simulink model "DynamicModel_DiferentialDrive"  (R2018a)
settings: Solver=ode4  StartTime=0.0  StopTime=100  FixedStep=0.01  RelTol=1e-3
libraries: simulink x1
settings Model: Creator=Yuri  LastModifiedBy=Yuri
settings SolverCC: AlgebraicLoopSolver=LineSearch

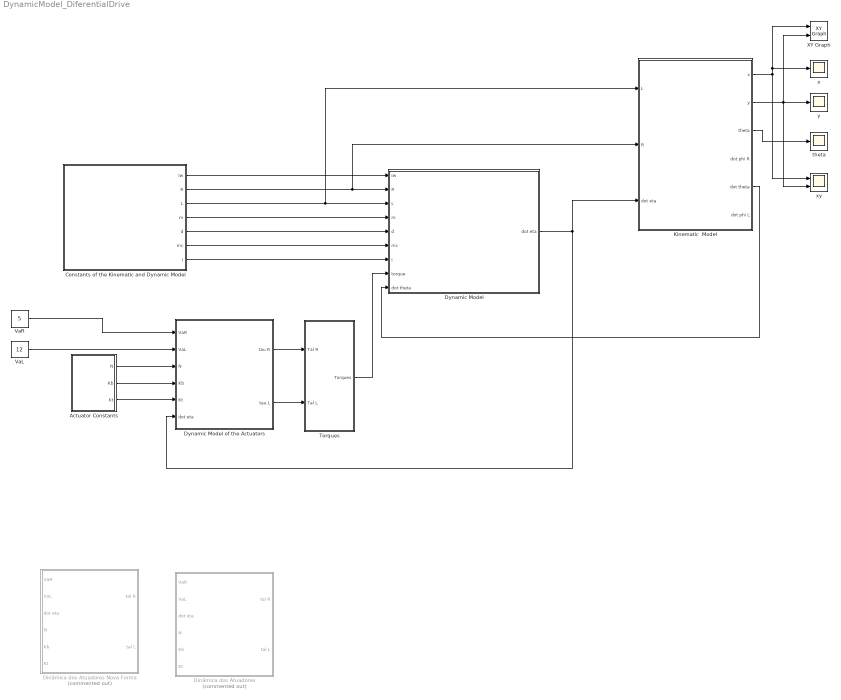
== system DynamicModel_DiferentialDrive ==
  Actuator Constants : Subsystem
  Constants of the Kinematic and Dynamic Model : Subsystem
  "Dinâmica dos Atuadores " : Subsystem  Commented=on
  Dinâmica dos Atuadores Nova Forma : Subsystem  Commented=on
  Dynamic Model : Subsystem
  Dynamic Model of the Actuators : Subsystem
  Kinematic  Model : Subsystem
  Torques : Subsystem
  VaL : Constant  Value=12
  VaR : Constant  Value=5
  XY Graph : simulink/Sinks/XY Graph  xmin=-25  xmax=25  ymin=-25  ymax=25  st=-1
  "theta " : Scope
  x : Scope
  xy : Scope  NumInputPorts=2
  y : Scope
  wires:
  Torques/1("Torques ") -> Dynamic Model/8(torque)
  Kinematic  Model/3(theta) -> "theta "/1
  Kinematic  Model/1(x) -> xy/1, XY Graph/1, x/1
  Kinematic  Model/2(y) -> xy/2, XY Graph/2, y/1
  Kinematic  Model/5(dot theta) -> Dynamic Model/9(dot theta)
  Dynamic Model/1(dot eta) -> Dynamic Model of the Actuators/6(dot eta), Kinematic  Model/3(dot eta)
  VaR/1 -> Dynamic Model of the Actuators/1(VaR)
  VaL/1 -> Dynamic Model of the Actuators/2(VaL)
  Dynamic Model of the Actuators/1(tau R) -> Torques/1(Tal R)
  Dynamic Model of the Actuators/2(tau L) -> Torques/2(Tal L)
  Constants of the Kinematic and Dynamic Model/5("d ") -> Dynamic Model/5(d)
  Constants of the Kinematic and Dynamic Model/3("L ") -> Kinematic  Model/1(L), Dynamic Model/3(L)
  Constants of the Kinematic and Dynamic Model/2("R ") -> Kinematic  Model/2(R), Dynamic Model/2(R)
  Constants of the Kinematic and Dynamic Model/6("mc ") -> Dynamic Model/6(mc)
  Constants of the Kinematic and Dynamic Model/1("Iw ") -> Dynamic Model/1(Iw)
  Constants of the Kinematic and Dynamic Model/4("m ") -> Dynamic Model/4(m)
  Actuator Constants/1(N) -> Dynamic Model of the Actuators/3("N ")
  Actuator Constants/3("Kt ") -> Dynamic Model of the Actuators/5("Kt ")
  Actuator Constants/2("Kb ") -> Dynamic Model of the Actuators/4("Kb ")
  Constants of the Kinematic and Dynamic Model/7("I ") -> Dynamic Model/7(I)

== system DynamicModel_DiferentialDrive/Actuator Constants ==
  Kb : Constant  Value=0.029
  Kt : Constant  Value=0.023
  "N  " : Constant  Value=38.3
  N : Outport
  "Kb " : Outport  Port=2
  "Kt " : Outport  Port=3
  wires:
  Kb/1 -> "Kb "/1
  Kt/1 -> "Kt "/1
  "N  "/1 -> N/1

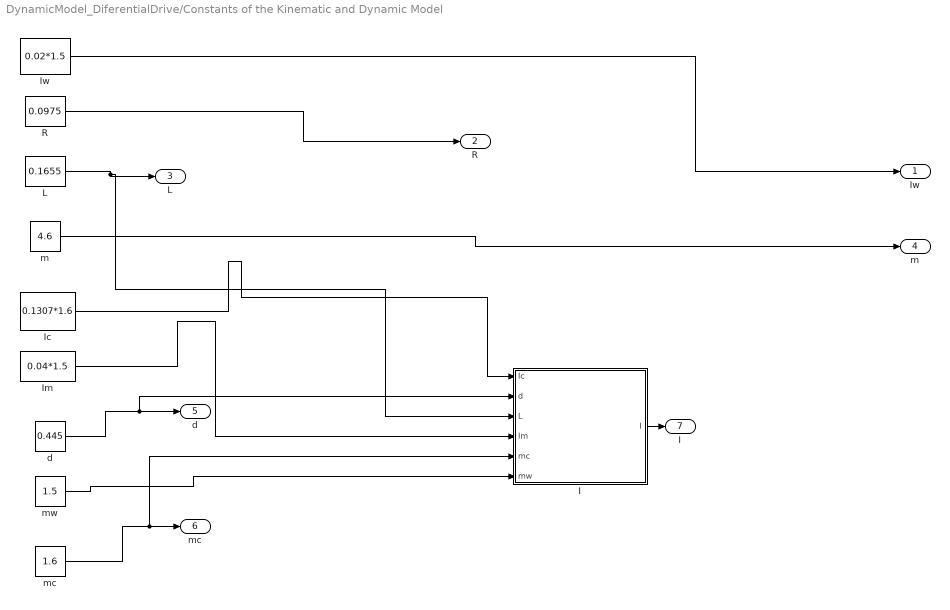
== system DynamicModel_DiferentialDrive/Constants of the Kinematic and Dynamic Model ==
  I : Subsystem
  Ic : Constant  Value=0.1307*1.6
  Im : Constant  Value=0.04*1.5
  Iw : Constant  Value=0.02*1.5
  L : Constant  Value=0.1655  VectorParams1D=off
  R : Constant  Value=0.0975
  d : Constant  Value=0.445
  m : Constant  Value=4.6
  mc : Constant  Value=1.6
  mw : Constant  Value=1.5
  "Iw " : Outport
  "R " : Outport  Port=2
  "L " : Outport  Port=3
  "m " : Outport  Port=4
  "d " : Outport  Port=5
  "mc " : Outport  Port=6
  "I " : Outport  Port=7
  wires:
  Im/1 -> I/4(Im)
  Ic/1 -> I/1(Ic)
  d/1 -> I/2(d), "d "/1
  R/1 -> "R "/1
  Iw/1 -> "Iw "/1
  mw/1 -> I/6(mw)
  m/1 -> "m "/1
  mc/1 -> I/5(mc), "mc "/1
  L/1 -> I/3(L), "L "/1
  I/1(I) -> "I "/1

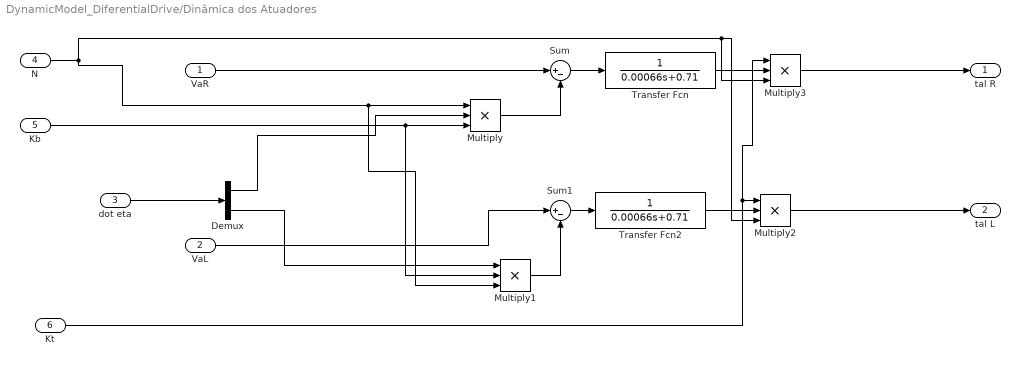
== system DynamicModel_DiferentialDrive/Dinâmica dos Atuadores  ==
  VaR : Inport
  VaL : Inport  Port=2
  dot eta : Inport  Port=3
  "N " : Inport  Port=4
  "Kb " : Inport  Port=5
  "Kt " : Inport  Port=6
  Demux : Demux  Outputs=2
  Multiply{,1..3} (4 alike) : Product  Inputs=3
  Sum : Sum  Inputs=|+-
  Sum1 : Sum  Inputs=|+-
  Transfer Fcn : TransferFcn  Denominator=[0.00066 0.71]
  Transfer Fcn2 : TransferFcn  Denominator=[0.00066 0.71]
  tal R : Outport
  tal L : Outport  Port=2
  wires:
  VaR/1 -> Sum/1
  Sum/1 -> Transfer Fcn/1
  Demux/1 -> Multiply/2
  VaL/1 -> Sum1/1
  Sum1/1 -> Transfer Fcn2/1
  Multiply1/1 -> Sum1/2
  dot eta/1 -> Demux/1
  "N "/1 -> Multiply1/3, Multiply/1, Multiply2/3, Multiply3/3
  "Kb "/1 -> Multiply1/2, Multiply/3
  Demux/2 -> Multiply1/1
  Multiply/1 -> Sum/2
  Transfer Fcn2/1 -> Multiply2/2
  Transfer Fcn/1 -> Multiply3/2
  "Kt "/1 -> Multiply3/1, Multiply2/1
  Multiply3/1 -> tal R/1
  Multiply2/1 -> tal L/1

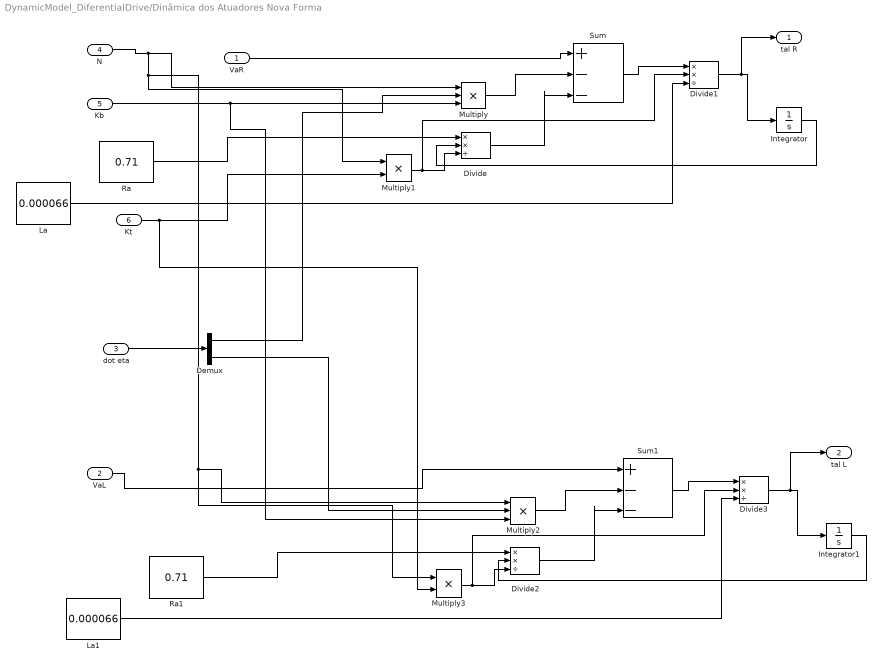
== system DynamicModel_DiferentialDrive/Dinâmica dos Atuadores Nova Forma ==
  VaR : Inport
  VaL : Inport  Port=2
  dot eta : Inport  Port=3
  "N " : Inport  Port=4
  "Kb " : Inport  Port=5
  "Kt " : Inport  Port=6
  Demux : Demux  Outputs=2
  Divide{,1..3} (4 alike) : Product  Inputs=**/
  Integrator : Integrator
  Integrator1 : Integrator
  La : Constant  Value=0.000066
  La1 : Constant  Value=0.000066
  Multiply : Product  Inputs=3
  Multiply1 : Product
  Multiply2 : Product  Inputs=3
  Multiply3 : Product
  Ra : Constant  Value=0.71
  Ra1 : Constant  Value=0.71
  Sum : Sum  Inputs=|+--
  Sum1 : Sum  Inputs=|+--
  tal R : Outport
  tal L : Outport  Port=2
  wires:
  VaR/1 -> Sum/1
  Demux/1 -> Multiply/2
  dot eta/1 -> Demux/1
  Multiply/1 -> Sum/2
  "Kt "/1 -> Multiply3/2, Multiply1/2
  Ra/1 -> Divide/1
  Multiply1/1 -> Divide1/2, Divide/3
  Integrator/1 -> Divide/2
  Divide/1 -> Sum/3
  Divide1/1 -> tal R/1, Integrator/1
  Sum/1 -> Divide1/1
  La/1 -> Divide1/3
  Divide3/1 -> tal L/1, Integrator1/1
  VaL/1 -> Sum1/1
  Demux/2 -> Multiply2/2
  Sum1/1 -> Divide3/1
  Multiply2/1 -> Sum1/2
  Divide2/1 -> Sum1/3
  "Kb "/1 -> Multiply2/3, Multiply/3
  Ra1/1 -> Divide2/1
  Integrator1/1 -> Divide2/2
  "N "/1 -> Multiply3/1, Multiply2/1, Multiply1/1, Multiply/1
  La1/1 -> Divide3/3
  Multiply3/1 -> Divide3/2, Divide2/3

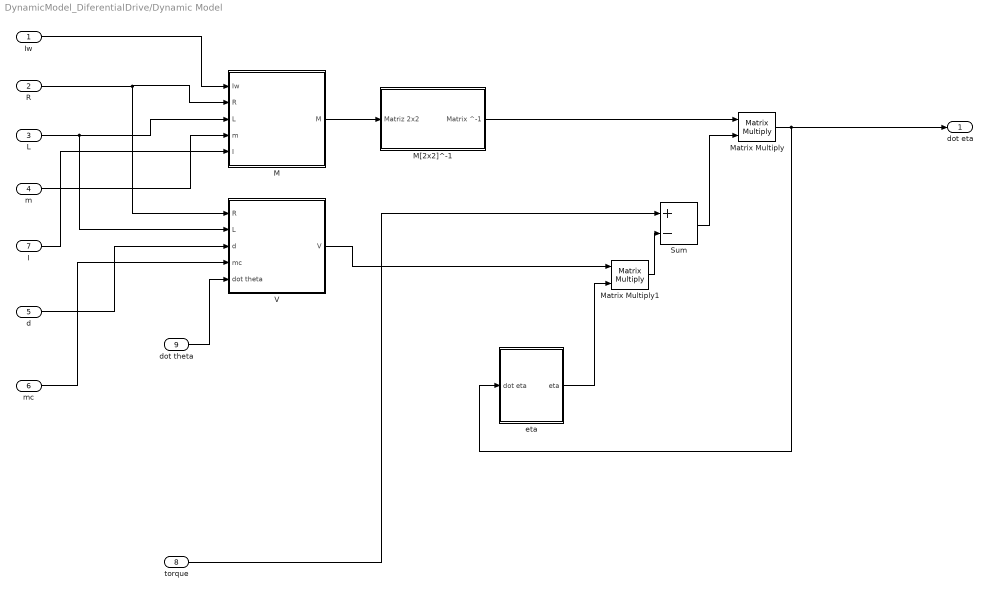
== system DynamicModel_DiferentialDrive/Dynamic Model ==
  Iw : Inport
  R : Inport  Port=2
  L : Inport  Port=3
  m : Inport  Port=4
  d : Inport  Port=5
  mc : Inport  Port=6
  I : Inport  Port=7
  torque : Inport  Port=8
  dot theta : Inport  Port=9
  " eta" : Subsystem
  M : Subsystem
  M[2x2]^-1 : Subsystem
  Matrix Multiply : Product  Multiplication=Matrix(*)
  Matrix Multiply1 : Product  Multiplication=Matrix(*)
  Sum : Sum  Inputs=+-
  V : Subsystem
  dot eta : Outport
  wires:
  Matrix Multiply1/1 -> Sum/2
  Sum/1 -> Matrix Multiply/2
  " eta"/1("eta ") -> Matrix Multiply1/2
  M[2x2]^-1/1(Matrix ^-1) -> Matrix Multiply/1
  Matrix Multiply/1 -> " eta"/1(dot eta), dot eta/1
  torque/1 -> Sum/1
  L/1 -> V/2(L), M/3(L)
  mc/1 -> V/4(mc)
  R/1 -> M/2(R), V/1(R)
  dot theta/1 -> V/5(dot theta)
  Iw/1 -> M/1(Iw)
  I/1 -> M/5(I)
  m/1 -> M/4(m)
  d/1 -> V/3(d)
  M/1(M) -> M[2x2]^-1/1("Matriz 2x2 ")
  V/1(V) -> Matrix Multiply1/1

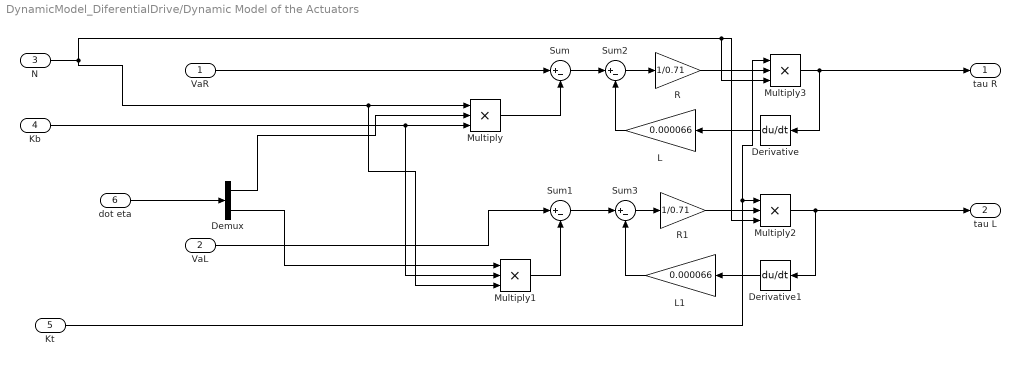
== system DynamicModel_DiferentialDrive/Dynamic Model of the Actuators ==
  VaR : Inport
  VaL : Inport  Port=2
  "N " : Inport  Port=3
  "Kb " : Inport  Port=4
  "Kt " : Inport  Port=5
  dot eta : Inport  Port=6
  Demux : Demux  Outputs=2
  Derivative : Derivative
  Derivative1 : Derivative
  L : Gain  Gain=0.000066
  L1 : Gain  Gain=0.000066
  Multiply{,1..3} (4 alike) : Product  Inputs=3
  R : Gain  Gain=1/0.71
  R1 : Gain  Gain=1/0.71
  Sum{,1..3} (4 alike) : Sum  Inputs=|+-
  tau R : Outport
  tau L : Outport  Port=2
  wires:
  VaR/1 -> Sum/1
  Sum/1 -> Sum2/1
  Demux/1 -> Multiply/2
  VaL/1 -> Sum1/1
  Multiply1/1 -> Sum1/2
  dot eta/1 -> Demux/1
  "N "/1 -> Multiply1/3, Multiply/1, Multiply2/3, Multiply3/3
  "Kb "/1 -> Multiply1/2, Multiply/3
  Demux/2 -> Multiply1/1
  Multiply/1 -> Sum/2
  R1/1 -> Multiply2/2
  Sum2/1 -> R/1
  "Kt "/1 -> Multiply3/1, Multiply2/1
  Multiply3/1 -> Derivative/1, tau R/1
  Multiply2/1 -> Derivative1/1, tau L/1
  Derivative/1 -> L/1
  L/1 -> Sum2/2
  R/1 -> Multiply3/2
  Sum3/1 -> R1/1
  Sum1/1 -> Sum3/1
  L1/1 -> Sum3/2
  Derivative1/1 -> L1/1

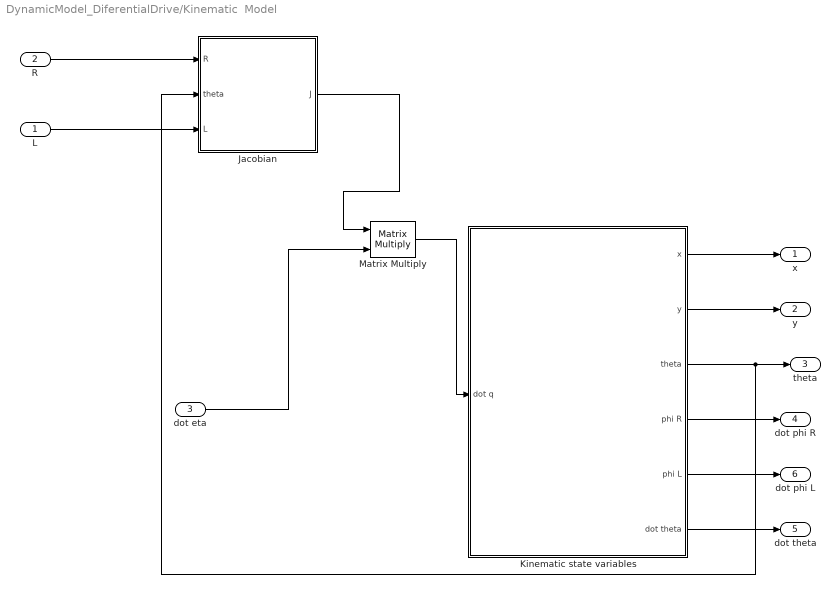
== system DynamicModel_DiferentialDrive/Kinematic  Model ==
  L : Inport
  R : Inport  Port=2
  dot eta : Inport  Port=3
  "Jacobian " : Subsystem
  Kinematic state variables : Subsystem
  Matrix Multiply : Product  Multiplication=Matrix(*)
  x : Outport
  y : Outport  Port=2
  theta : Outport  Port=3
  dot phi R : Outport  Port=4
  dot theta : Outport  Port=5
  dot phi L : Outport  Port=6
  wires:
  Matrix Multiply/1 -> Kinematic state variables/1("dot q ")
  "Jacobian "/1(J) -> Matrix Multiply/1
  Kinematic state variables/5(phi L) -> dot phi L/1
  Kinematic state variables/1(x) -> x/1
  Kinematic state variables/3(theta) -> theta/1, "Jacobian "/2(theta)
  Kinematic state variables/6(dot theta) -> dot theta/1
  R/1 -> "Jacobian "/1(R)
  Kinematic state variables/4(phi R) -> dot phi R/1
  Kinematic state variables/2(y) -> y/1
  L/1 -> "Jacobian "/3(L)
  dot eta/1 -> Matrix Multiply/2

== system DynamicModel_DiferentialDrive/Torques ==
  Tal R : Inport
  Tal L : Inport  Port=2
  Mux : Mux  Inputs=2
  "[2,1]" : Reshape  OutputDimensionality=Customize  OutputDimensions=[2,1]
  "Torques " : Outport
  wires:
  Tal R/1 -> Mux/1
  Tal L/1 -> Mux/2
  Mux/1 -> "[2,1]"/1
  "[2,1]"/1 -> "Torques "/1

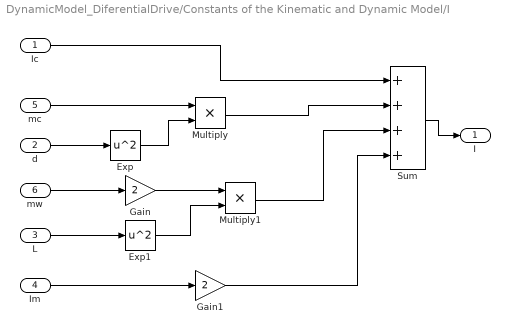
== system DynamicModel_DiferentialDrive/Constants of the Kinematic and Dynamic Model/I ==
  Ic : Inport
  d : Inport  Port=2
  L : Inport  Port=3
  Im : Inport  Port=4
  mc : Inport  Port=5
  mw : Inport  Port=6
  Exp : Math  Operator=square  SaturateOnIntegerOverflow=on
  Exp1 : Math  Operator=square  SaturateOnIntegerOverflow=on
  Gain : Gain  Gain=2
  Gain1 : Gain  Gain=2
  Multiply : Product
  Multiply1 : Product
  Sum : Sum  Inputs=++++
  I : Outport
  wires:
  Ic/1 -> Sum/1
  d/1 -> Exp/1
  Exp/1 -> Multiply/2
  mc/1 -> Multiply/1
  Multiply/1 -> Sum/2
  L/1 -> Exp1/1
  mw/1 -> Gain/1
  Exp1/1 -> Multiply1/2
  Gain/1 -> Multiply1/1
  Multiply1/1 -> Sum/3
  Im/1 -> Gain1/1
  Gain1/1 -> Sum/4
  Sum/1 -> I/1

== system DynamicModel_DiferentialDrive/Dynamic Model/ eta ==
  dot eta : Inport
  Demux : Demux  Outputs=2
  Integrator : Integrator
  Integrator1 : Integrator
  Mux : Mux  Inputs=2
  "[2,1]" : Reshape  OutputDimensionality=Customize  OutputDimensions=[2,1]
  "eta " : Outport
  wires:
  dot eta/1 -> Demux/1
  Demux/1 -> Integrator/1
  Demux/2 -> Integrator1/1
  Integrator1/1 -> Mux/2
  Integrator/1 -> Mux/1
  Mux/1 -> "[2,1]"/1
  "[2,1]"/1 -> "eta "/1

== system DynamicModel_DiferentialDrive/Dynamic Model/M ==
  Iw : Inport
  R : Inport  Port=2
  L : Inport  Port=3
  m : Inport  Port=4
  I : Inport  Port=5
  M11 e M22 : Subsystem
  M12 e M21 : Subsystem
  Mux1 : Mux
  "[1x4] to [2,2]" : Reshape  OutputDimensionality=Customize  OutputDimensions=[2,2]
  M : Outport
  wires:
  Iw/1 -> M11 e M22/1(Iw)
  Mux1/1 -> "[1x4] to [2,2]"/1
  R/1 -> M12 e M21/1(R), M11 e M22/2(R)
  L/1 -> M12 e M21/2(L), M11 e M22/3(L)
  m/1 -> M12 e M21/3("m "), M11 e M22/4("m ")
  I/1 -> M12 e M21/4(I), M11 e M22/5(I)
  M11 e M22/1(M11) -> Mux1/4, Mux1/1
  M12 e M21/1(M12) -> Mux1/3, Mux1/2
  "[1x4] to [2,2]"/1 -> M/1

== system DynamicModel_DiferentialDrive/Dynamic Model/M[2x2]^-1 ==
  "Matriz 2x2 " : Inport
  Demux : Demux
  Gain : Gain  Gain=-1
  Gain1 : Gain  Gain=-1
  Mux : Mux
  Reshape : Reshape  OutputDimensionality=Customize  OutputDimensions=[4,1]
  Reshape1 : Reshape  OutputDimensionality=Customize  OutputDimensions=[2,2]
  Matrix ^-1 : Outport
  wires:
  "Matriz 2x2 "/1 -> Reshape/1
  Demux/1 -> Mux/4
  Demux/4 -> Mux/1
  Demux/2 -> Gain/1
  Gain/1 -> Mux/2
  Demux/3 -> Gain1/1
  Gain1/1 -> Mux/3
  Mux/1 -> Reshape1/1
  Reshape/1 -> Demux/1
  Reshape1/1 -> Matrix ^-1/1

== system DynamicModel_DiferentialDrive/Dynamic Model/V ==
  R : Inport
  L : Inport  Port=2
  d : Inport  Port=3
  mc : Inport  Port=4
  dot theta : Inport  Port=5
  Constant : Constant  Value=0
  Mux1 : Mux
  V12 : Subsystem
  V21 : Subsystem
  "[4x1] to [2,2]" : Reshape  OutputDimensionality=Customize  OutputDimensions=[2,2]
  V : Outport
  wires:
  Constant/1 -> Mux1/4, Mux1/1
  V12/1("V12 ") -> Mux1/2
  V21/1("V21 ") -> Mux1/3
  R/1 -> V21/1(R), V12/1(R)
  L/1 -> V21/2(L), V12/2(L)
  d/1 -> V21/3(d), V12/3(d)
  dot theta/1 -> V21/5(dot theta), V12/5(dot theta)
  mc/1 -> V21/4(mc), V12/4(mc)
  Mux1/1 -> "[4x1] to [2,2]"/1
  "[4x1] to [2,2]"/1 -> V/1

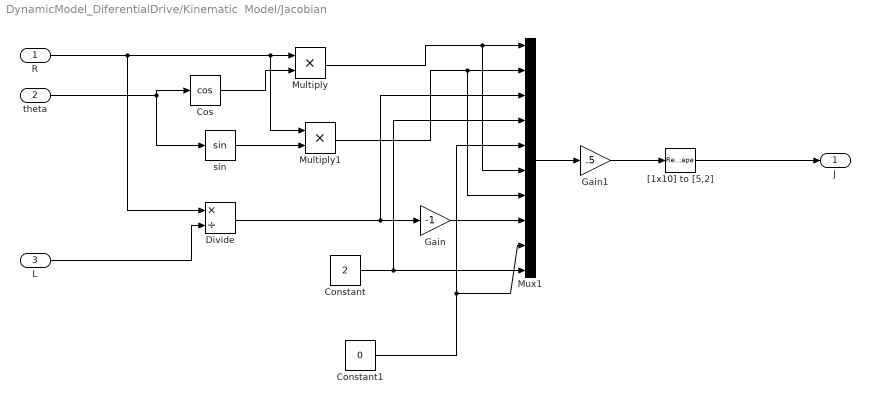
== system DynamicModel_DiferentialDrive/Kinematic  Model/Jacobian  ==
  R : Inport
  theta : Inport  Port=2
  L : Inport  Port=3
  Constant : Constant  Value=2
  Constant1 : Constant  Value=0
  Cos : Trigonometry  Operator=cos
  Divide : Product  Inputs=*/
  Gain : Gain  Gain=-1
  Gain1 : Gain  Gain=.5
  Multiply : Product
  Multiply1 : Product
  Mux1 : Mux  Inputs=10
  "[1x10] to [5,2]" : Reshape  OutputDimensionality=Customize  OutputDimensions=[5,2]
  sin : Trigonometry
  J : Outport
  wires:
  R/1 -> Divide/1, Multiply1/1, Multiply/1
  L/1 -> Divide/2
  Mux1/1 -> Gain1/1
  theta/1 -> sin/1, Cos/1
  Cos/1 -> Multiply/2
  Multiply/1 -> Mux1/6, Mux1/1
  sin/1 -> Multiply1/2
  Divide/1 -> Mux1/3, Gain/1
  Constant/1 -> Mux1/4, Mux1/10
  "[1x10] to [5,2]"/1 -> J/1
  Gain1/1 -> "[1x10] to [5,2]"/1
  Multiply1/1 -> Mux1/7, Mux1/2
  Constant1/1 -> Mux1/9, Mux1/5
  Gain/1 -> Mux1/8

== system DynamicModel_DiferentialDrive/Kinematic  Model/Kinematic state variables ==
  "dot q " : Inport
  " q" : Subsystem
  dot q : Subsystem
  theta1 : Subsystem
  x : Outport
  y : Outport  Port=2
  theta : Outport  Port=3
  phi R : Outport  Port=4
  phi L : Outport  Port=5
  dot theta : Outport  Port=6
  wires:
  dot q/1(dot x) -> " q"/1(dot x)
  dot q/4(dot phi R) -> " q"/4(dot phi R)
  dot q/3(dot theta) -> dot theta/1, " q"/3(dot theta)
  dot q/5(dot phi L) -> " q"/5(dot phi L)
  dot q/2(dot y) -> " q"/2(dot y)
  " q"/5(" phi L") -> phi L/1
  "dot q "/1 -> dot q/1(dot q)
  " q"/4(" phi R") -> phi R/1
  " q"/1(" x") -> x/1
  " q"/2(" y") -> y/1
  " q"/3(" theta") -> theta1/1(theta)
  theta1/1(theta [-pi,pi]) -> theta/1

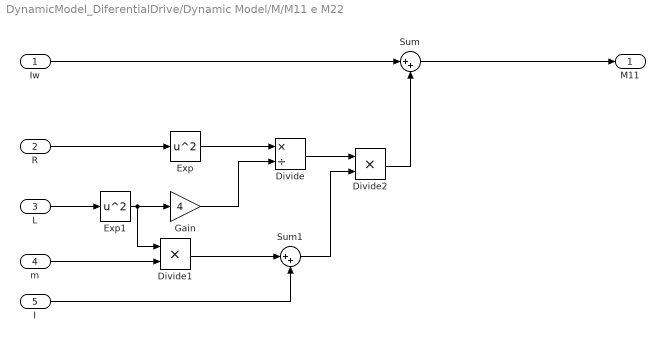
== system DynamicModel_DiferentialDrive/Dynamic Model/M/M11 e M22 ==
  Iw : Inport
  R : Inport  Port=2
  L : Inport  Port=3
  "m " : Inport  Port=4
  I : Inport  Port=5
  Divide : Product  Inputs=*/
  Divide1 : Product  Inputs=**
  Divide2 : Product  Inputs=**
  Exp : Math  Operator=square  SaturateOnIntegerOverflow=on
  Exp1 : Math  Operator=square  SaturateOnIntegerOverflow=on
  Gain : Gain  Gain=4
  Sum : Sum  Inputs=|++
  Sum1 : Sum  Inputs=|++
  M11 : Outport
  wires:
  Iw/1 -> Sum/1
  Sum/1 -> M11/1
  R/1 -> Exp/1
  Exp/1 -> Divide/1
  L/1 -> Exp1/1
  Exp1/1 -> Divide1/1, Gain/1
  Gain/1 -> Divide/2
  "m "/1 -> Divide1/2
  Divide1/1 -> Sum1/1
  I/1 -> Sum1/2
  Divide/1 -> Divide2/1
  Sum1/1 -> Divide2/2
  Divide2/1 -> Sum/2

== system DynamicModel_DiferentialDrive/Dynamic Model/M/M12 e M21 ==
  R : Inport
  L : Inport  Port=2
  "m " : Inport  Port=3
  I : Inport  Port=4
  Divide : Product  Inputs=*/
  Divide1 : Product  Inputs=**
  Divide2 : Product  Inputs=**
  Exp : Math  Operator=square  SaturateOnIntegerOverflow=on
  Exp1 : Math  Operator=square  SaturateOnIntegerOverflow=on
  Gain : Gain  Gain=4
  Sum1 : Sum  Inputs=|+-
  M12 : Outport
  wires:
  Divide2/1 -> M12/1
  R/1 -> Exp/1
  Exp/1 -> Divide/1
  L/1 -> Exp1/1
  Exp1/1 -> Divide1/1, Gain/1
  Gain/1 -> Divide/2
  "m "/1 -> Divide1/2
  Divide1/1 -> Sum1/1
  I/1 -> Sum1/2
  Divide/1 -> Divide2/1
  Sum1/1 -> Divide2/2

== system DynamicModel_DiferentialDrive/Dynamic Model/V/V12 ==
  R : Inport
  L : Inport  Port=2
  d : Inport  Port=3
  mc : Inport  Port=4
  dot theta : Inport  Port=5
  Divide : Product  Inputs=*/
  Exp : Math  Operator=square  SaturateOnIntegerOverflow=on
  Gain : Gain  Gain=2
  Multiply : Product
  Multiply1 : Product
  Multiply2 : Product
  "V12 " : Outport
  wires:
  Exp/1 -> Divide/1
  L/1 -> Gain/1
  Gain/1 -> Divide/2
  R/1 -> Exp/1
  Divide/1 -> Multiply/1
  d/1 -> Multiply/2
  mc/1 -> Multiply1/1
  dot theta/1 -> Multiply1/2
  Multiply2/1 -> "V12 "/1
  Multiply/1 -> Multiply2/1
  Multiply1/1 -> Multiply2/2

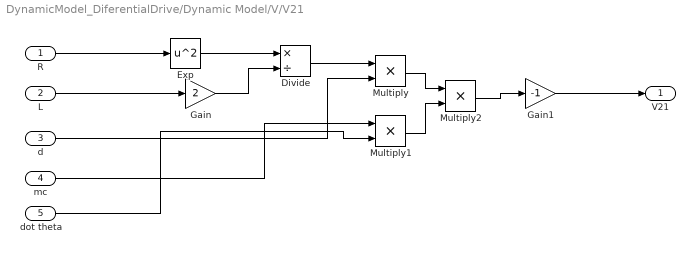
== system DynamicModel_DiferentialDrive/Dynamic Model/V/V21 ==
  R : Inport
  L : Inport  Port=2
  d : Inport  Port=3
  mc : Inport  Port=4
  dot theta : Inport  Port=5
  Divide : Product  Inputs=*/
  Exp : Math  Operator=square  SaturateOnIntegerOverflow=on
  Gain : Gain  Gain=2
  Gain1 : Gain  Gain=-1
  Multiply : Product
  Multiply1 : Product
  Multiply2 : Product
  "V21 " : Outport
  wires:
  Exp/1 -> Divide/1
  L/1 -> Gain/1
  Gain/1 -> Divide/2
  R/1 -> Exp/1
  Divide/1 -> Multiply/1
  d/1 -> Multiply/2
  mc/1 -> Multiply1/1
  dot theta/1 -> Multiply1/2
  Multiply2/1 -> Gain1/1
  Gain1/1 -> "V21 "/1
  Multiply1/1 -> Multiply2/2
  Multiply/1 -> Multiply2/1

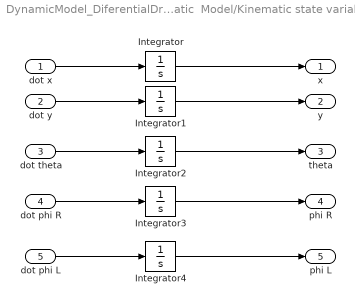
== system DynamicModel_DiferentialDrive/Kinematic  Model/Kinematic state variables/ q ==
  dot x : Inport
  dot y : Inport  Port=2
  dot theta : Inport  Port=3
  dot phi R : Inport  Port=4
  dot phi L : Inport  Port=5
  Integrator{,1..4} (5 alike) : Integrator
  " x" : Outport
  " y" : Outport  Port=2
  " theta" : Outport  Port=3
  " phi R" : Outport  Port=4
  " phi L" : Outport  Port=5
  wires:
  dot x/1 -> Integrator/1
  Integrator/1 -> " x"/1
  dot y/1 -> Integrator1/1
  Integrator1/1 -> " y"/1
  dot theta/1 -> Integrator2/1
  Integrator2/1 -> " theta"/1
  dot phi R/1 -> Integrator3/1
  Integrator3/1 -> " phi R"/1
  dot phi L/1 -> Integrator4/1
  Integrator4/1 -> " phi L"/1

== system DynamicModel_DiferentialDrive/Kinematic  Model/Kinematic state variables/dot q ==
  dot q : Inport
  Demux : Demux  Outputs=5
  dot x : Outport
  dot y : Outport  Port=2
  dot theta : Outport  Port=3
  dot phi R : Outport  Port=4
  dot phi L : Outport  Port=5
  wires:
  Demux/2 -> dot y/1
  dot q/1 -> Demux/1
  Demux/1 -> dot x/1
  Demux/3 -> dot theta/1
  Demux/4 -> dot phi R/1
  Demux/5 -> dot phi L/1

== system DynamicModel_DiferentialDrive/Kinematic  Model/Kinematic state variables/theta1 ==
  theta : Inport
  Atan2 : Trigonometry  Operator=atan2
  Cos : Trigonometry  Operator=cos
  Sin : Trigonometry
  theta [-pi,pi] : Outport
  wires:
  theta/1 -> Cos/1, Sin/1
  Atan2/1 -> theta [-pi,pi]/1
  Sin/1 -> Atan2/1
  Cos/1 -> Atan2/2
